simulink model "recursive_arimax_model_update"  (R2020a)
settings: Solver=FixedStepAuto  StartTime=1944  StopTime=1970  FixedStep=1  RelTol=1e-3
settings Model: Creator=tyoshida  LastModifiedBy=tyoshida

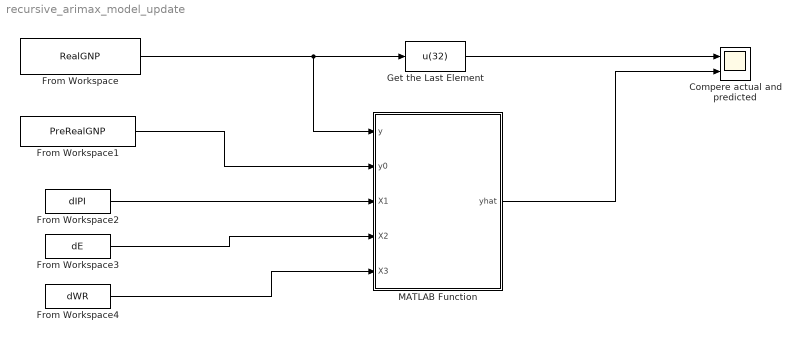
== system recursive_arimax_model_update ==
  Compere actual and predicted : Scope  NumInputPorts=2
  From Workspace : FromWorkspace  VariableName=RealGNP
  From Workspace1 : FromWorkspace  VariableName=PreRealGNP
  From Workspace2 : FromWorkspace  VariableName=dIPI
  From Workspace3 : FromWorkspace  VariableName=dE
  From Workspace4 : FromWorkspace  VariableName=dWR
  Get the Last Element : Fcn  Expr=u(32)
  MATLAB Function : MATLAB Function  TreatAsAtomicUnit=on
  wires:
  From Workspace/1 -> Get the Last Element/1, MATLAB Function/1(y)
  From Workspace1/1 -> MATLAB Function/2(y0)
  MATLAB Function/1(yhat) -> Compere actual and predicted/2
  Get the Last Element/1 -> Compere actual and predicted/1
  From Workspace2/1 -> MATLAB Function/3(X1)
  From Workspace3/1 -> MATLAB Function/4(X2)
  From Workspace4/1 -> MATLAB Function/5(X3)

== matlab function recursive_arimax_model_update/MATLAB Function ==
  data: y input; yhat output; y0 input; X1 input; X2 input; X3 input
function yhat = ARIMAX_Predictor(y, y0, X1, X2, X3)

yhat = 0; % WA because the analyzer cannot identify this data type for code generation

Degree = [2,1,2];
X = [X1,X2,X3];
coder.extrinsic('my_arimax_predict_fcn'); % declare extrinsic functions for code generation
yhat = my_arimax_predict_fcn(Degree, y(1:end-1), y0, X);

end
